simulink model "Lab6"  (R2019a)
settings: Solver=VariableStepAuto  StartTime=0.0  StopTime=12  RelTol=1e-3
values from neighbouring files (symbols this model uses):
  atan_scale = 100    [test1.mat]
  b_1 = 0.00287081256979    [test1.mat]
  b_2 = 0.000164101446955    [test1.mat]
  b_3 = 0.000179179608867    [test1.mat]
  C = [1 0 0 0 0 0 0 1 0 0 0 0 ... (18 elements, 3x6)]    [test1.mat]
  f_m = [0 -0.025 0]    [test1.mat]
  J_1 = 0.00238607064451    [test1.mat]
  J_2 = 0.00182883419357    [test1.mat]
  J_3 = 0.00182883419357    [test1.mat]
  k_1 = 2.78736928639    [test1.mat]
  k_2 = 2.53389832968    [test1.mat]
  T_Cm = 0.0969711017207    [test1.mat]
  T_Cp = 0.0714454263135    [test1.mat]
  T_s = 0.004    [test1.mat]
  w_th = 0.75    [test1.mat]
  x_0 = [0 0 0 0 0 0]    [test1.mat]
undefined symbols (not defined in the file or in its folder): G_y1_d, G_y2_d, G_y3_d, h_sol, mu_0, mu_1_sol, sigma_1, var_r0, wn, zeta
settings Model: Creator=Ian  LastModifiedBy=Ian

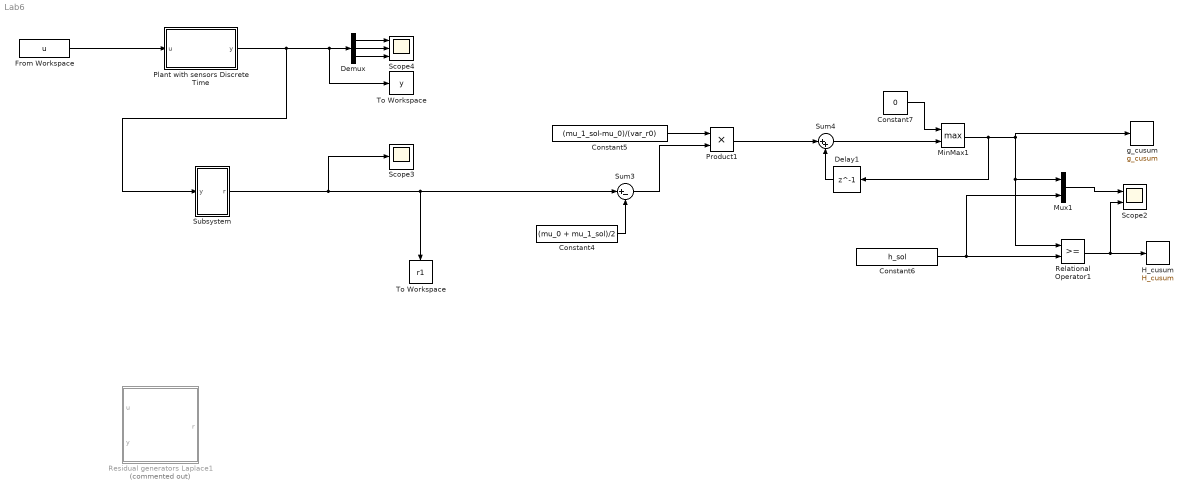
== system Lab6 ==
  Constant4 : Constant  Value=(mu_0 + mu_1_sol)/2
  Constant5 : Constant  Value=(mu_1_sol-mu_0)/(var_r0)
  Constant6 : Constant  Value=h_sol  VectorParams1D=off
  Constant7 : Constant  Value=0
  Delay1 : Delay  DelayLength=1  SampleTime=0.004
  Demux : Demux  Outputs=3
  From Workspace : FromWorkspace  VariableName=u  SampleTime=0
  H_cusum : ToWorkspace  VariableName=H_cusum  SaveFormat=Structure With Time  SampleTime=-1
  MinMax1 : MinMax  Function=max  Inputs=2
  Mux1 : Mux  Inputs=2
  Plant with sensors Discrete Time : Subsystem
  Product1 : Product
  Relational Operator1 : RelationalOperator  OutDataTypeStr=boolean  RndMeth=Simplest
  Residual generators Laplace1 : Subsystem  Commented=on
  Scope2 : Scope  NumInputPorts=2
  Scope3 : Scope
  Scope4 : Scope  NumInputPorts=3
  Subsystem : Subsystem
  Sum3 : Sum  Inputs=|+-
  Sum4 : Sum  Inputs=|++
  To Workspace : ToWorkspace  VariableName=y  SaveFormat=Structure With Time  SampleTime=-1
  "To Workspace " : ToWorkspace  VariableName=r1  SaveFormat=Structure With Time  SampleTime=-1
  g_cusum : ToWorkspace  VariableName=g_cusum  SaveFormat=Structure With Time  SampleTime=-1
  wires:
  Relational Operator1/1 -> H_cusum/1, Scope2/2
  Constant6/1 -> Mux1/2, Relational Operator1/2
  Subsystem/1(r) -> Scope3/1, Sum3/1, "To Workspace "/1
  Plant with sensors Discrete Time/1(y) -> Subsystem/1(y), To Workspace/1, Demux/1
  Constant5/1 -> Product1/1
  From Workspace/1 -> Plant with sensors Discrete Time/1(u)
  Demux/1 -> Scope4/1
  Delay1/1 -> Sum4/2
  Demux/3 -> Scope4/3
  Constant4/1 -> Sum3/2
  Mux1/1 -> Scope2/1
  Constant7/1 -> MinMax1/1
  Demux/2 -> Scope4/2
  MinMax1/1 -> Delay1/1, g_cusum/1, Mux1/1, Relational Operator1/1
  Product1/1 -> Sum4/1
  Sum4/1 -> MinMax1/2
  Sum3/1 -> Product1/2

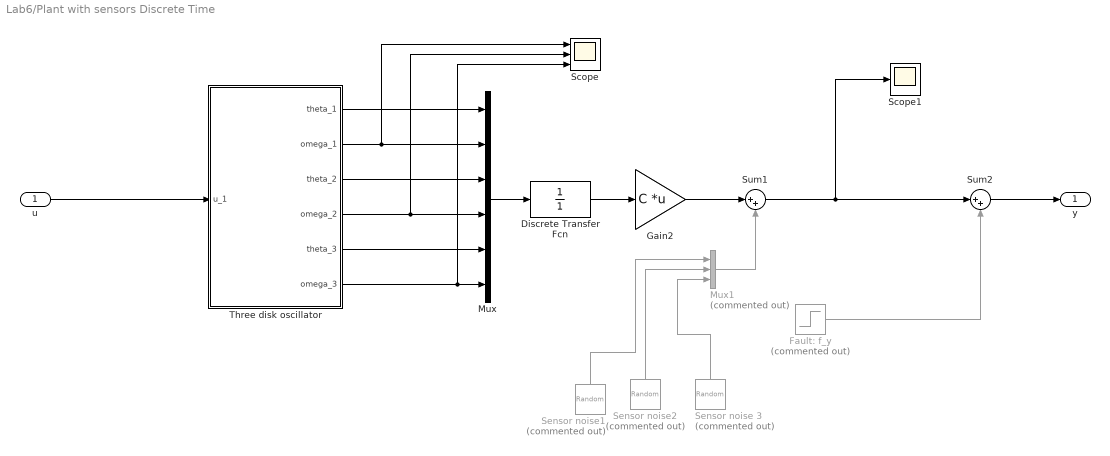
== system Lab6/Plant with sensors Discrete Time ==
  u : Inport
  Discrete Transfer Fcn : DiscreteTransferFcn  Denominator=[1]  SampleTime=0.004
  Fault: f_y : Step  Commented=on  Time=8.5  Before=[0;0;0]  After=[0;f_m;0]  SampleTime=0
  Gain2 : Gain  Gain=C  Multiplication=Matrix(K*u) (u vector)
  Mux : Mux  Inputs=6
  Mux1 : Mux  Commented=on  Inputs=3
  Scope : Scope  NumInputPorts=3
  Scope1 : Scope
  Sensor noise 3 : RandomNumber  Commented=on  Variance=0.01^2  Seed=2159  SampleTime=T_s
  Sensor noise1 : RandomNumber  Commented=on  Variance=0.01^2  Seed=215924  SampleTime=T_s
  Sensor noise2 : RandomNumber  Commented=on  Variance=0.01^2  Seed=21524  SampleTime=T_s
  Sum1 : Sum  Inputs=|++
  Sum2 : Sum  Inputs=|++
  Three disk oscillator : Subsystem
  y : Outport
  wires:
  u/1 -> Three disk oscillator/1(u_1)
  Three disk oscillator/2(omega_1) -> Scope/1, Mux/2
  Three disk oscillator/1(theta_1) -> Mux/1
  Mux/1 -> Discrete Transfer Fcn/1
  Three disk oscillator/4(omega_2) -> Scope/2, Mux/4
  Three disk oscillator/3(theta_2) -> Mux/3
  Discrete Transfer Fcn/1 -> Gain2/1
  Sum2/1 -> y/1
  Three disk oscillator/6(omega_3) -> Scope/3, Mux/6
  Three disk oscillator/5(theta_3) -> Mux/5
  Sum1/1 -> Scope1/1, Sum2/1
  Gain2/1 -> Sum1/1
  Fault: f_y/1 -> Sum2/2
  Sensor noise1/1 -> Mux1/1
  Sensor noise2/1 -> Mux1/2
  Sensor noise 3/1 -> Mux1/3
  Mux1/1 -> Sum1/2

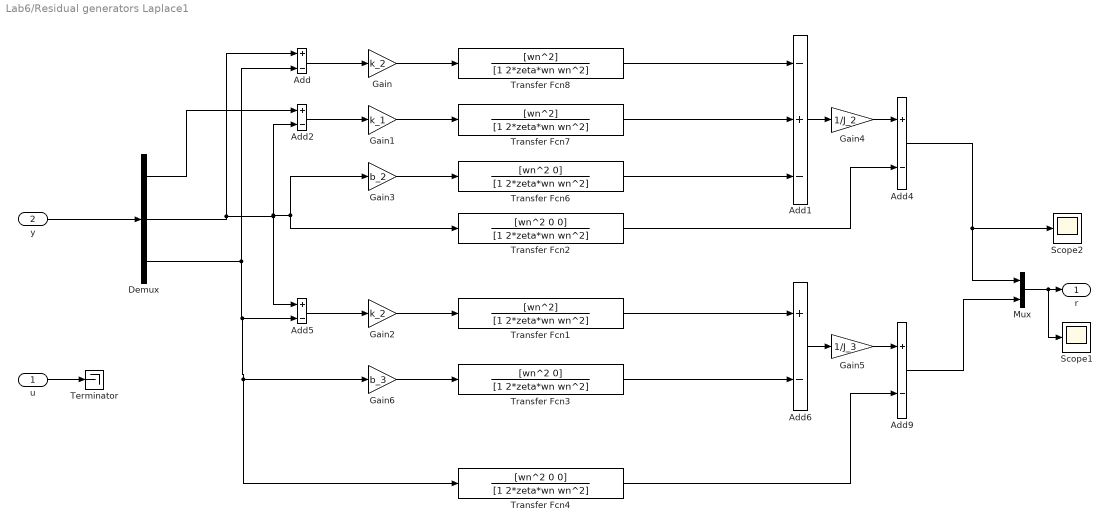
== system Lab6/Residual generators Laplace1 ==
  u : Inport
  y : Inport  Port=2
  Add{,2,4..6,9} (6 alike) : Sum  Inputs=+-
  Add1 : Sum  Inputs=-+-
  Demux : Demux  Outputs=3
  Gain : Gain  Gain=k_2
  Gain1 : Gain  Gain=k_1
  Gain2 : Gain  Gain=k_2
  Gain3 : Gain  Gain=b_2
  Gain4 : Gain  Gain=1/J_2
  Gain5 : Gain  Gain=1/J_3
  Gain6 : Gain  Gain=b_3
  Mux : Mux  Inputs=2
  Scope1 : Scope
  Scope2 : Scope
  Terminator : Terminator
  Transfer Fcn1 : TransferFcn  Numerator=[wn^2]  Denominator=[1 2*zeta*wn wn^2]
  Transfer Fcn2 : TransferFcn  Numerator=[wn^2 0 0]  Denominator=[1 2*zeta*wn wn^2]
  Transfer Fcn3 : TransferFcn  Numerator=[wn^2 0]  Denominator=[1 2*zeta*wn wn^2]
  Transfer Fcn4 : TransferFcn  Numerator=[wn^2 0 0]  Denominator=[1 2*zeta*wn wn^2]
  Transfer Fcn6 : TransferFcn  Numerator=[wn^2 0]  Denominator=[1 2*zeta*wn wn^2]
  Transfer Fcn7 : TransferFcn  Numerator=[wn^2]  Denominator=[1 2*zeta*wn wn^2]
  Transfer Fcn8 : TransferFcn  Numerator=[wn^2]  Denominator=[1 2*zeta*wn wn^2]
  r : Outport
  wires:
  y/1 -> Demux/1
  u/1 -> Terminator/1
  Add/1 -> Gain/1
  Add2/1 -> Gain1/1
  Add1/1 -> Gain4/1
  Gain4/1 -> Add4/1
  Demux/2 -> Add5/1, Transfer Fcn2/1, Gain3/1, Add2/2, Add/1
  Add5/1 -> Gain2/1
  Add6/1 -> Gain5/1
  Gain5/1 -> Add9/1
  Demux/1 -> Add2/1
  Gain6/1 -> Transfer Fcn3/1
  Demux/3 -> Transfer Fcn4/1, Gain6/1, Add5/2, Add/2
  Mux/1 -> Scope1/1, r/1
  Add4/1 -> Mux/1, Scope2/1
  Add9/1 -> Mux/2
  Transfer Fcn2/1 -> Add4/2
  Gain/1 -> Transfer Fcn8/1
  Gain1/1 -> Transfer Fcn7/1
  Transfer Fcn8/1 -> Add1/1
  Gain2/1 -> Transfer Fcn1/1
  Transfer Fcn7/1 -> Add1/2
  Gain3/1 -> Transfer Fcn6/1
  Transfer Fcn6/1 -> Add1/3
  Transfer Fcn1/1 -> Add6/1
  Transfer Fcn3/1 -> Add6/2
  Transfer Fcn4/1 -> Add9/2

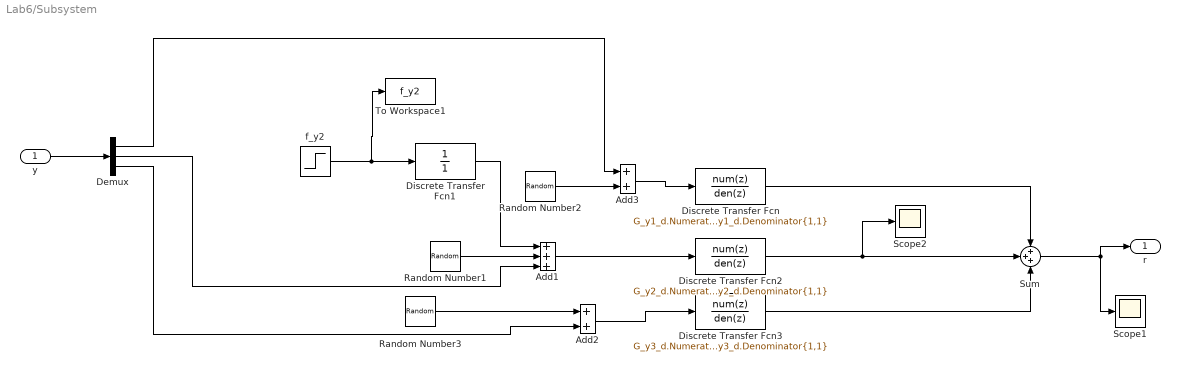
== system Lab6/Subsystem ==
  y : Inport
  Add1 : Sum  Inputs=+++
  Add2 : Sum
  Add3 : Sum
  Demux : Demux  Outputs=3
  Discrete Transfer Fcn : DiscreteTransferFcn  Numerator=G_y1_d.Numerator{1,1}  Denominator=G_y1_d.Denominator{1,1}
  Discrete Transfer Fcn1 : DiscreteTransferFcn  Denominator=[1]  SampleTime=0.004
  Discrete Transfer Fcn2 : DiscreteTransferFcn  Numerator=G_y2_d.Numerator{1,1}  Denominator=G_y2_d.Denominator{1,1}
  Discrete Transfer Fcn3 : DiscreteTransferFcn  Numerator=G_y3_d.Numerator{1,1}  Denominator=G_y3_d.Denominator{1,1}
  Random Number1 : RandomNumber  Variance=sigma_1^2  Seed=2137  SampleTime=T_s
  Random Number2 : RandomNumber  Variance=sigma_1^2  Seed=1242  SampleTime=T_s
  Random Number3 : RandomNumber  Variance=sigma_1^2  Seed=2434923  SampleTime=T_s
  Scope1 : Scope
  Scope2 : Scope
  Sum : Sum  Inputs=+++
  To Workspace1 : ToWorkspace  VariableName=f_y2  SaveFormat=Structure With Time  SampleTime=-1
  "f_y2 " : Step  Time=8.5  After=f_m  SampleTime=0
  r : Outport
  wires:
  Sum/1 -> r/1, Scope1/1
  Add1/1 -> Discrete Transfer Fcn2/1
  "f_y2 "/1 -> Discrete Transfer Fcn1/1, To Workspace1/1
  Discrete Transfer Fcn2/1 -> Scope2/1, Sum/2
  Discrete Transfer Fcn/1 -> Sum/1
  Random Number1/1 -> Add1/2
  Discrete Transfer Fcn3/1 -> Sum/3
  y/1 -> Demux/1
  Demux/2 -> Add1/3
  Random Number3/1 -> Add2/1
  Demux/3 -> Add2/2
  Add2/1 -> Discrete Transfer Fcn3/1
  Random Number2/1 -> Add3/2
  Add3/1 -> Discrete Transfer Fcn/1
  Demux/1 -> Add3/1
  Discrete Transfer Fcn1/1 -> Add1/1

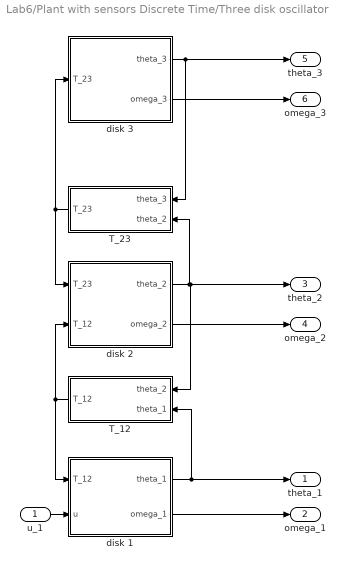
== system Lab6/Plant with sensors Discrete Time/Three disk oscillator ==
  u_1 : Inport
  T_12 : Subsystem
  T_23 : Subsystem
  disk 1 : Subsystem
  disk 2 : Subsystem
  disk 3 : Subsystem
  theta_1 : Outport
  omega_1 : Outport  Port=2
  theta_2 : Outport  Port=3
  omega_2 : Outport  Port=4
  theta_3 : Outport  Port=5
  omega_3 : Outport  Port=6
  wires:
  T_23/1(T_23) -> disk 2/1(T_23), disk 3/1(T_23)
  disk 1/1(theta_1) -> T_12/2(theta_1), theta_1/1
  disk 2/1(theta_2) -> T_23/2(theta_2), theta_2/1, T_12/1(theta_2)
  T_12/1(T_12) -> disk 1/1(T_12), disk 2/2(T_12)
  disk 3/2(omega_3) -> omega_3/1
  disk 1/2(omega_1) -> omega_1/1
  disk 2/2(omega_2) -> omega_2/1
  u_1/1 -> disk 1/2(u)
  disk 3/1(theta_3) -> theta_3/1, T_23/1(theta_3)

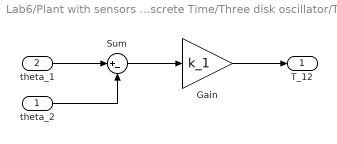
== system Lab6/Plant with sensors Discrete Time/Three disk oscillator/T_12 ==
  theta_2 : Inport
  theta_1 : Inport  Port=2
  Gain : Gain  Gain=k_1
  Sum : Sum  Inputs=|+-
  T_12 : Outport
  wires:
  theta_2/1 -> Sum/2
  theta_1/1 -> Sum/1
  Sum/1 -> Gain/1
  Gain/1 -> T_12/1

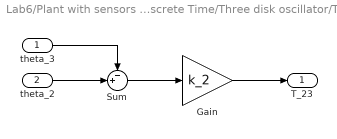
== system Lab6/Plant with sensors Discrete Time/Three disk oscillator/T_23 ==
  theta_3 : Inport
  theta_2 : Inport  Port=2
  Gain : Gain  Gain=k_2
  Sum : Sum  Inputs=-+|
  T_23 : Outport
  wires:
  Gain/1 -> T_23/1
  Sum/1 -> Gain/1
  theta_3/1 -> Sum/1
  theta_2/1 -> Sum/2

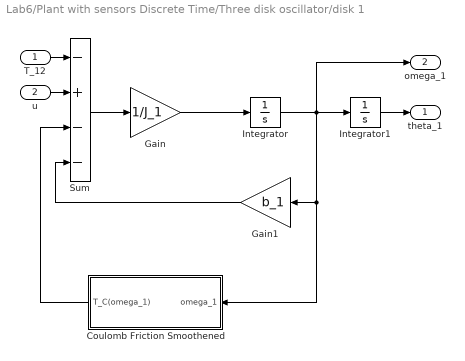
== system Lab6/Plant with sensors Discrete Time/Three disk oscillator/disk 1 ==
  T_12 : Inport
  u : Inport  Port=2
  Coulomb Friction Smoothened : Subsystem
  Gain : Gain  Gain=1/J_1
  Gain1 : Gain  Gain=b_1
  Integrator : Integrator  InitialCondition=x_0(2)
  Integrator1 : Integrator  InitialCondition=x_0(1)
  Sum : Sum  Inputs=-+--
  theta_1 : Outport
  omega_1 : Outport  Port=2
  wires:
  Sum/1 -> Gain/1
  Integrator/1 -> Integrator1/1, omega_1/1, Coulomb Friction Smoothened/1(omega_1), Gain1/1
  Gain1/1 -> Sum/4
  Integrator1/1 -> theta_1/1
  T_12/1 -> Sum/1
  u/1 -> Sum/2
  Gain/1 -> Integrator/1
  Coulomb Friction Smoothened/1(T_C(omega_1)) -> Sum/3

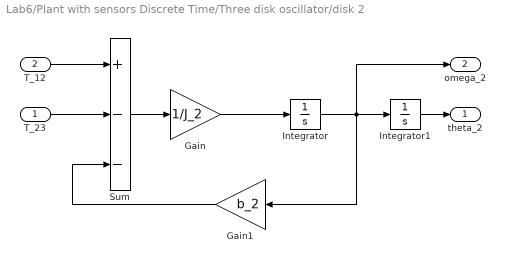
== system Lab6/Plant with sensors Discrete Time/Three disk oscillator/disk 2 ==
  T_23 : Inport
  T_12 : Inport  Port=2
  Gain : Gain  Gain=1/J_2
  Gain1 : Gain  Gain=b_2
  Integrator : Integrator  InitialCondition=x_0(4)
  Integrator1 : Integrator  InitialCondition=x_0(3)
  Sum : Sum  Inputs=+--
  theta_2 : Outport
  omega_2 : Outport  Port=2
  wires:
  T_23/1 -> Sum/2
  T_12/1 -> Sum/1
  Integrator1/1 -> theta_2/1
  Gain1/1 -> Sum/3
  Gain/1 -> Integrator/1
  Integrator/1 -> Integrator1/1, Gain1/1, omega_2/1
  Sum/1 -> Gain/1

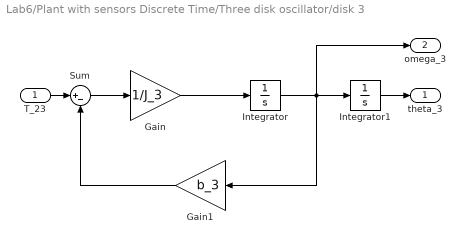
== system Lab6/Plant with sensors Discrete Time/Three disk oscillator/disk 3 ==
  T_23 : Inport
  Gain : Gain  Gain=1/J_3
  Gain1 : Gain  Gain=b_3
  Integrator : Integrator  InitialCondition=x_0(6)
  Integrator1 : Integrator  InitialCondition=x_0(5)
  Sum : Sum  Inputs=|+-
  theta_3 : Outport
  omega_3 : Outport  Port=2
  wires:
  Sum/1 -> Gain/1
  Integrator/1 -> Integrator1/1, omega_3/1, Gain1/1
  Gain/1 -> Integrator/1
  Gain1/1 -> Sum/2
  Integrator1/1 -> theta_3/1
  T_23/1 -> Sum/1

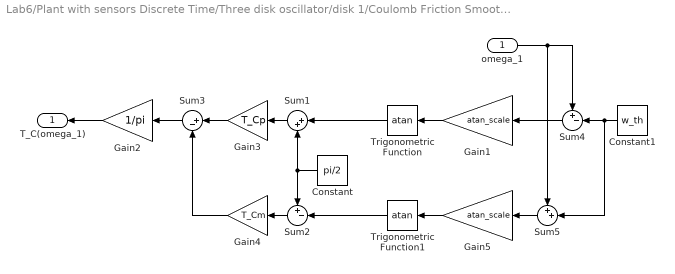
== system Lab6/Plant with sensors Discrete Time/Three disk oscillator/disk 1/Coulomb Friction Smoothened ==
  omega_1 : Inport
  Constant : Constant  Value=pi/2
  Constant1 : Constant  Value=w_th
  Gain1 : Gain  Gain=atan_scale
  Gain2 : Gain  Gain=1/pi
  Gain3 : Gain  Gain=T_Cp
  Gain4 : Gain  Gain=T_Cm
  Gain5 : Gain  Gain=atan_scale
  Sum1 : Sum  Inputs=|++
  Sum2 : Sum  Inputs=+-|
  Sum3 : Sum  Inputs=|+-
  Sum4 : Sum  Inputs=+-|
  Sum5 : Sum  Inputs=++|
  Trigonometric Function : Trigonometry  Operator=atan
  Trigonometric Function1 : Trigonometry  Operator=atan
  T_C(omega_1) : Outport
  wires:
  Gain1/1 -> Trigonometric Function/1
  Sum1/1 -> Gain3/1
  Constant/1 -> Sum2/1, Sum1/2
  Sum2/1 -> Gain4/1
  Sum3/1 -> Gain2/1
  Trigonometric Function/1 -> Sum1/1
  Gain4/1 -> Sum3/2
  Gain2/1 -> T_C(omega_1)/1
  omega_1/1 -> Sum5/1, Sum4/1
  Gain3/1 -> Sum3/1
  Sum4/1 -> Gain1/1
  Constant1/1 -> Sum5/2, Sum4/2
  Gain5/1 -> Trigonometric Function1/1
  Sum5/1 -> Gain5/1
  Trigonometric Function1/1 -> Sum2/2
